simulink model "neodnorodni"  (Simulink 7.9)
settings: Solver=ode45  StartTime=-10.0  StopTime=100.0  RelTol=1e-3
libraries: simulink x1
settings Model: Creator=Mihail  LastModifiedBy=Mihail

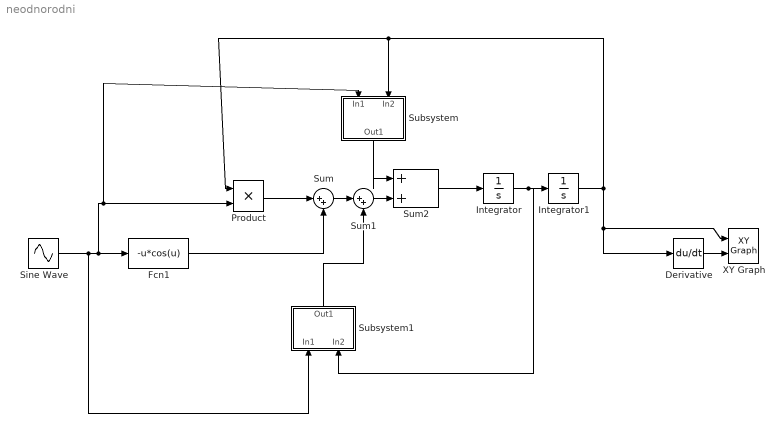
== system neodnorodni ==
  Derivative : Derivative
  Fcn1 : Fcn  Expr=-u*cos(u)
  Integrator : Integrator
  Integrator1 : Integrator
  Product : Product  RndMeth=Zero
  Sine Wave : Sin  SampleTime=0
  Subsystem : Subsystem
  Subsystem1 : Subsystem
  Sum : Sum  Inputs=|++
  Sum1 : Sum  Inputs=|++
  Sum2 : Sum  Inputs=|++
  XY Graph : simulink/Sinks/XY Graph  xmin=-1  xmax=1  ymin=-1  ymax=1  st=-1
  wires:
  Sine Wave/1 -> Fcn1/1, Product/2, Subsystem/1(In1), Subsystem1/1(In1)
  Product/1 -> Sum/1
  Fcn1/1 -> Sum/2
  Sum/1 -> Sum1/1
  Integrator1/1 -> XY Graph/1, Derivative/1, Product/1, Subsystem/2(In2)
  Derivative/1 -> XY Graph/2
  Integrator/1 -> Integrator1/1, Subsystem1/2(In2)
  Sum2/1 -> Integrator/1
  Subsystem1/1(Out1) -> Sum1/2
  Sum1/1 -> Sum2/2
  Subsystem/1(Out1) -> Sum2/1

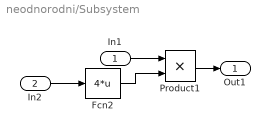
== system neodnorodni/Subsystem ==
  In1 : Inport
  In2 : Inport  Port=2
  Fcn2 : Fcn  Expr=4*u
  Product1 : Product  RndMeth=Zero
  Out1 : Outport
  wires:
  Fcn2/1 -> Product1/2
  In1/1 -> Product1/1
  In2/1 -> Fcn2/1
  Product1/1 -> Out1/1

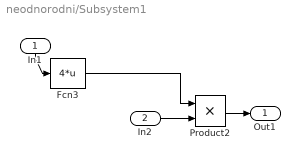
== system neodnorodni/Subsystem1 ==
  In1 : Inport
  In2 : Inport  Port=2
  Fcn3 : Fcn  Expr=4*u
  Product2 : Product  RndMeth=Zero
  Out1 : Outport
  wires:
  Fcn3/1 -> Product2/1
  In1/1 -> Fcn3/1
  In2/1 -> Product2/2
  Product2/1 -> Out1/1
